simulink model "Glideslope_control"  (R2023a)
settings: Solver=ode5  StartTime=0.0  StopTime=20  FixedStep=0.001  RelTol=1e-3  EnableMultiTasking=on
values from neighbouring files (symbols this model uses):
  trim_control_lin = trim_control_lo    [CAP_Gipson_Criterion.m]    (also in FindF16Dynamics.m; Glideslope.m; ali_glidslope.m; openloop.m)
  trim_thrust_lin = trim_thrust_lo    [CAP_Gipson_Criterion.m]    (also in FindF16Dynamics.m; Glideslope.m; ali_glidslope.m; openloop.m)
libraries: cstblocks x1
settings Model: Creator=keviczky  LastModifiedBy=anape
settings SolverCC: AlgebraicLoopSolver=TrustRegion
settings DataIOCC: Decimation=50  SaveFormat=Array  SignalLoggingSaveFormat=ModelDataLogs  ReturnWorkspaceOutputs=off  SignalLoggingName=sigsOut
settings OptimizationCC: BooleanDataType=off
settings DebuggingCC: SaveWithParameterizedLinksMsg=none  UnderspecifiedInitializationDetection=Classic  MergeDetectMultiDrivingBlocksExec=none  SignalResolutionControl=TryResolveAllWithWarning  MultiTaskDSMMsg=warning  MultiTaskCondExecSysMsg=none  UnconnectedInputMsg=warning  UnconnectedOutputMsg=warning  UnconnectedLineMsg=warning
settings HardwareCC: ProdBitPerPointer=32  ProdBitPerSizeT=32  ProdBitPerPtrDiffT=32  ProdLargestAtomicFloat=None  ProdIntDivRoundTo=Undefined  ProdEndianess=Unspecified  ProdWordSize=32  ProdHWDeviceType=32-bit Generic  TargetUnknown=on
settings ModelReferenceCC: EnableRefExpFcnMdlSchedulingChecks=on  PropagateSignalLabelsOutOfModel=off
settings RTWCC: DLArmComputeVersion=19.05
settings GRTTargetCC: CombineOutputUpdateFcns=off  GRTInterface=on
settings ConfigComp: CovMetricSettings=dw  CovSaveCumulativeToWorkspaceVar=on  CovSaveSingleToWorkspaceVar=on

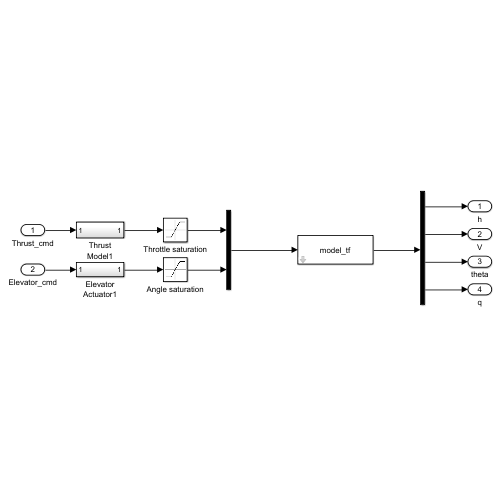
[thumbnail: Simulink's stored preview of the top-level diagram]
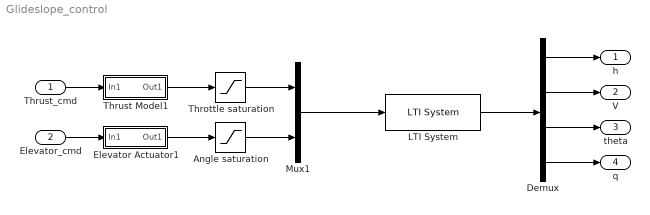
== system Glideslope_control ==
  Thrust_cmd : Inport
  Elevator_cmd : Inport  Port=2
  Angle saturation : Saturate  UpperLimit=25  LowerLimit=-25
  Demux : Demux
  Elevator Actuator1 : Subsystem  AncestorBlock=F16_Actuator_Library/Elevator Actuator
      settings: LibrarySourceBlock=|
      | F16_Actuator_Library/Elevator
      | Actuator
  LTI System : cstblocks/LTI System  sys=model_tf  IC=[]
  Mux1 : Mux  Inputs=2
  Throttle saturation : Saturate  UpperLimit=19000  LowerLimit=1000
  Thrust Model1 : Subsystem  AncestorBlock=F16_Actuator_Library/Thrust Model
      settings: LibrarySourceBlock=|
      | F16_Actuator_Library/Thrust
      | Model
  h : Outport
  V : Outport  Port=2
  theta : Outport  Port=3
  q : Outport  Port=4
  wires:
  Elevator_cmd/1 -> Elevator Actuator1/1(In1)
  Elevator Actuator1/1(Out1) -> Angle saturation/1
  Thrust Model1/1(Out1) -> Throttle saturation/1
  Thrust_cmd/1 -> Thrust Model1/1(In1)
  Throttle saturation/1 -> Mux1/1
  Angle saturation/1 -> Mux1/2
  Demux/1 -> h/1
  Demux/2 -> V/1
  Demux/3 -> theta/1
  Demux/4 -> q/1
  Mux1/1 -> LTI System/1
  LTI System/1 -> Demux/1

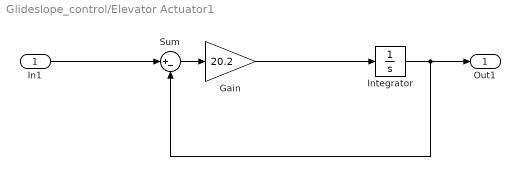
== system Glideslope_control/Elevator Actuator1 ==
  In1 : Inport
  Gain : Gain  Gain=20.2  SaturateOnIntegerOverflow=on  OutDataTypeStr=Inherit: Same as input  ParamDataTypeStr=Inherit: Same as input
  "Integrator " : Integrator  InitialCondition=trim_control_lin(1)  UpperSaturationLimit=25  LowerSaturationLimit=-25  ContinuousStateAttributes='elevator_state'
  Sum : Sum  Inputs=|+-  InputSameDT=on  SaturateOnIntegerOverflow=on  OutDataTypeStr=Inherit: Same as first input
  Out1 : Outport
  wires:
  "Integrator "/1 -> Sum/2, Out1/1
  Gain/1 -> "Integrator "/1
  Sum/1 -> Gain/1
  In1/1 -> Sum/1

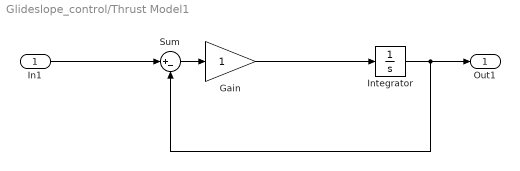
== system Glideslope_control/Thrust Model1 ==
  In1 : Inport
  Gain : Gain  SaturateOnIntegerOverflow=on  OutDataTypeStr=Inherit: Same as input  ParamDataTypeStr=Inherit: Same as input
  "Integrator " : Integrator  InitialCondition=trim_thrust_lin  UpperSaturationLimit=30  LowerSaturationLimit=-30  ContinuousStateAttributes='thrust_state'
  Sum : Sum  Inputs=|+-  InputSameDT=on  SaturateOnIntegerOverflow=on  OutDataTypeStr=Inherit: Same as first input
  Out1 : Outport
  wires:
  "Integrator "/1 -> Sum/2, Out1/1
  Gain/1 -> "Integrator "/1
  Sum/1 -> Gain/1
  In1/1 -> Sum/1
